simulink subsystem "hvb"  (R2020b)
settings: Solver=VariableStepAuto  StartTime=0.0  StopTime=10.0  RelTol=1e-3
undefined symbols (not defined in the file or in its folder): AmbTemp, batteryHV, DiscIntNeverNeededParam, hvBatterySOC_pct, motorDrive, nominalCapacity_kWh, packVoltage_V
libraries: fl_lib x14, nesl_utility x10, sdl_lib x1, ee_lib x1
settings Model: Creator=Dmitry  LastModifiedBy=Dmitry

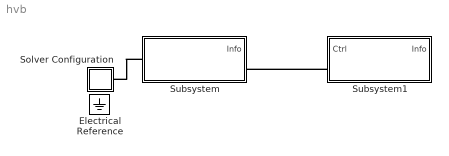
== system hvb ==
  Electrical Reference : fl_lib/Electrical/Electrical Elements/Electrical Reference
  Solver Configuration : Subsystem
      settings: PortSchema="{\"entries\":[{\"content\":{\"sides\":[{\"content\":{\"connectorIds\":[]},\"type\":\"ConnectorPlacement.EquallySpacedRectSide\",\"uuid\":\"4a7e26c2-e9e9-4fea-b605-533b1a682be7\"},{\"content\":{\"connectorIds\":[\"RConn1\"],\"side\":\"RIGHT\"},\"type\":\"ConnectorPlacement.EquallySpacedRectSide\",\"uuid\":\"0210e324-555e-4372-b836-fcc8ab23e933\"},{\"content\":{\"connectorIds\":[],\"side\":\"TOP\"},\"type\":\"ConnectorPlacement.EquallySpacedRectSide\",\"uuid\":\"9bbae011-e6fc-4534-a44f-d79a5697c939\"},{\"content\":{\"connectorIds\":[\"RConn2\"],\"side\":\"BOTTOM\"},\"type\":\"ConnectorPlacement.EquallySpacedRectSide\",\"uuid\":\"d5829c0a-26ea-402d-a1c6-900997ddf1a8\"}]},\"type\":\"ConnectorPlacement.EquallySpacedConnector\",\"uuid\":\"f4e17c65-54c6-42fe-a467-9c6b014b697a\"}],\"packageUris\":[\"http://schema.mathworks.com/mf0/Connector/19700101\"],\"version\":\"1.0\"}"
  Subsystem : Subsystem
  Subsystem1 : Subsystem
  connections:
  Subsystem/LConn1 -- Solver Configuration/RConn1
  Subsystem1/LConn1 -- Subsystem/RConn1

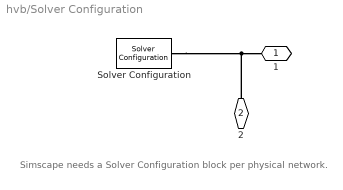
== system hvb/Solver Configuration ==
  note: Simscape needs a Solver Configuration block per physical network.
  Solver Configuration : nesl_utility/Solver Configuration  PhysicalDomain=network_engine_domain  SubClassName=solver  LeftPortType=input  RightPortType=generic  Tones=[]  Harmonics=[]  SimulateNoise=off  Profile=off  UseLocalSampling=off  EnableSwitchedLinearOptims=on  FrequencyDomain=off  UseCCode=off  RelTol=0.001  AbsTol=1e-06  MinStep=1e-09  ToWorkspace=off  RevertToSquareIcSolve=off  NumHomotopyIterations=100  PhasorMode=off  PhasorModeNumHarmonics=1  DoDC=off  ResidualTolerance=1e-6  UseLocalSolver=off  LocalSolverChoice=NE_BACKWARD_EULER_ADVANCER  LocalSolverSampleTime=0.01  DoFixedCost=off  MaxNonlinIter=3  MaxModeIter=2  ComputeImpulses=off  ImpulseIterations=2  LinearAlgebra=auto  EquationFormulation=NE_TIME_EF  DelaysMemoryBudget=1024  AutomaticFiltering=on  FilteringTimeConstant=0.001  PartitionStorageMethod=AS_NEEDED  PartitionMemoryBudget=1024  PartitionMethod=FAST
      settings: AttributesFormatString=Local solver %<UseLocalSolver>
  1 : PMIOPort  Side=Right
  2 : PMIOPort  Port=2  Side=Right
  connections:
  Solver Configuration/RConn1 -- 1/RConn1 -- 2/RConn1

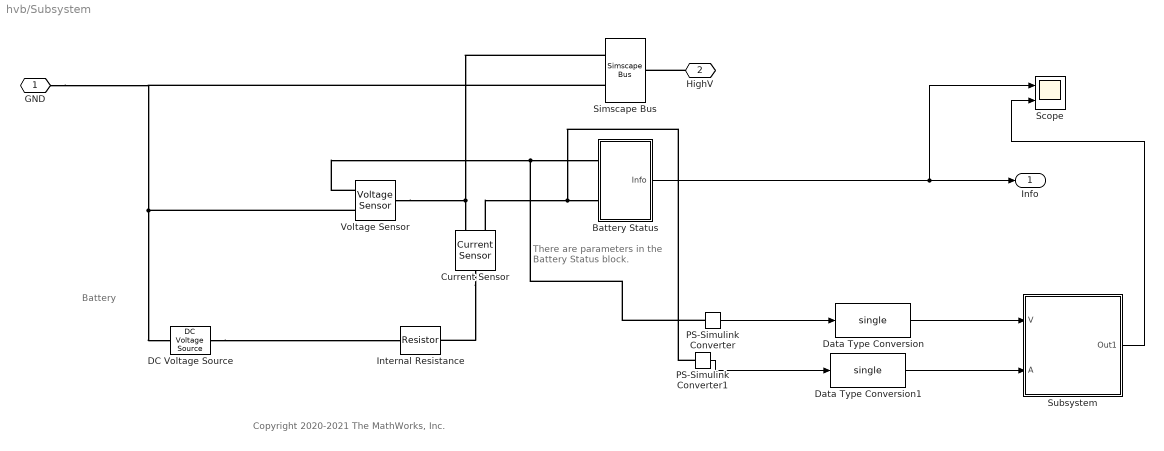
== system hvb/Subsystem ==
  note: Copyright 2020-2021 The MathWorks, Inc.
  note: There are parameters
      | in the Battery Status block.
  note: Battery
  Battery Status : Subsystem
  Current Sensor : fl_lib/Electrical/Electrical Sensors/Current Sensor
  DC Voltage Source : fl_lib/Electrical/Electrical Sources/DC Voltage Source  v0=batteryHV.packVoltage_V V
      settings: AttributesFormatString=%<v0> [%<v0_unit>]
  Data Type Conversion : DataTypeConversion  OutDataTypeStr=single
  Data Type Conversion1 : DataTypeConversion  OutDataTypeStr=single
  Internal Resistance : fl_lib/Electrical/Electrical Elements/Resistor  R=batteryHV.internal_R_Ohm Ohm  i_specify=off  i_priority=High  i=0 A  i_nominal_specify=off  i_nominal_unit=A  i_nominal_value=1  v_specify=off  v_priority=High  v=0 V  v_nominal_specify=off  v_nominal_unit=V  v_nominal_value=1
      settings: AttributesFormatString=%<R> [%<R_unit>]
  PS-Simulink Converter : nesl_utility/PS-Simulink Converter  PhysicalDomain=network_engine_domain  SubClassName=ps_output  LeftPortType=input  RightPortType=output  PseudoPeriodic=off  Frequencies=[]  Unit=inherit  AffineConversion=off
  PS-Simulink Converter1 : nesl_utility/PS-Simulink Converter  PhysicalDomain=network_engine_domain  SubClassName=ps_output  LeftPortType=input  RightPortType=output  PseudoPeriodic=off  Frequencies=[]  Unit=inherit  AffineConversion=off
  Scope : Scope  NumInputPorts=2
  Simscape Bus : SimscapeBus  HierarchyStrings=plus;minus
  Subsystem : Subsystem
  Voltage Sensor : fl_lib/Electrical/Electrical Sensors/Voltage Sensor
  GND : PMIOPort  Side=Left
  HighV : PMIOPort  Port=2  Side=Right
  Info : Outport
  wires:
  Data Type Conversion/1 -> Subsystem/1(V)
  PS-Simulink Converter1/1 -> Data Type Conversion1/1
  Battery Status/1(Info) -> Scope/1, Info/1
  Data Type Conversion1/1 -> Subsystem/2(A)
  PS-Simulink Converter/1 -> Data Type Conversion/1
  Subsystem/1(Out1) -> Scope/2
  connections:
  Voltage Sensor/RConn2 -- DC Voltage Source/RConn1 -- GND/RConn1 -- Simscape Bus/LConn2
  Simscape Bus/LConn1 -- Voltage Sensor/LConn1 -- Current Sensor/RConn2
  Current Sensor/RConn1 -- PS-Simulink Converter1/LConn1 -- Battery Status/LConn2
  Voltage Sensor/RConn1 -- PS-Simulink Converter/LConn1 -- Battery Status/LConn1
  HighV/RConn1 -- Simscape Bus/RConn1
  DC Voltage Source/LConn1 -- Internal Resistance/LConn1
  Current Sensor/LConn1 -- Internal Resistance/RConn1

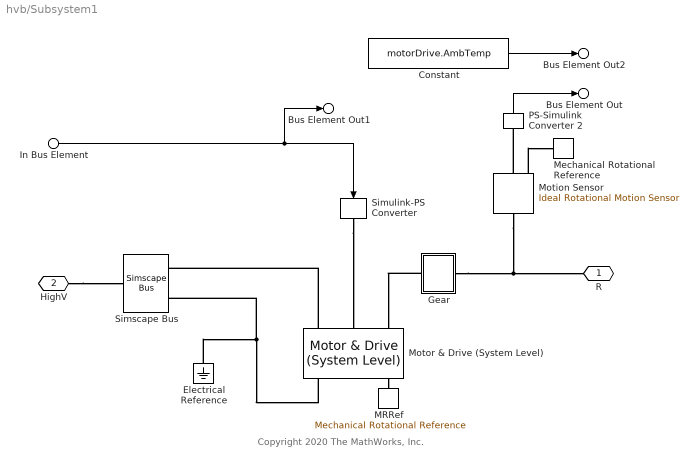
== system hvb/Subsystem1 ==
  note: Copyright 2020 The MathWorks, Inc.
  In Bus Element : Inport  PortName=Ctrl  Element=TorqueCmd
      settings: AttributesFormatString=%<Unit>
  " Simscape Bus" : SimscapeBus  HierarchyStrings=plus;minus
  Constant : Constant  Value=motorDrive.AmbTemp
  Electrical Reference : fl_lib/Electrical/Electrical Elements/Electrical Reference
  Gear : Subsystem
  MRRef : fl_lib/Mechanical/Rotational Elements/Mechanical Rotational Reference
  Mechanical Rotational Reference : fl_lib/Mechanical/Rotational Elements/Mechanical Rotational Reference
  Motion Sensor : fl_lib/Mechanical/Mechanical Sensors/Ideal Rotational Motion Sensor  wrap_angle=simscape.enum.onoff.off  offset=0 rad
  Motor & Drive (System Level) : ee_lib/Electromechanical/Motor & Drive (System Level)  torque_speed_param=2  overtorque_param=ee.enum.electromech.overtorque.no  T_t=[.09, .08, .07, 0] N*m  T_t_intermittent=[.36, .32, .28, 0] N*m  w_t=[0, 3750, 7500, 8000] rpm  torque_max=motorDrive.simplePmsmDrv_trqMax_Nm N*m  power_max=motorDrive.simplePmsmDrv_powMax_W W  torque_max_intermittent=0.4 N*m  power_max_intermittent=120 W  time_overtorque=30 s  time_recover=60 s  Tc=motorDrive.simplePmsmDrv_timeConst_s s  losses_param=2  eff=100  w_eff=3750 rpm  T_eff=0.08 N*m  Piron=0 W  Pbase=0 W  w_eff_vec=motorDrive.simplePmsmDrv_spdVec_rpm rpm  T_eff_vec=motorDrive.simplePmsmDrv_trqVec_Nm N*m  v_eff_vec=[100, 250, 400] V  losses_mat=motorDrive.simplePmsmDrv_LossTbl_W W  efficiency_mat=[95, 95, 95, 95; 95, 95, 95, 95; 95, 95, 95, 95; 95, 95, 95, 95; 95, 95, 95, 95]  losses_mat_3D=ones(5, 4, 3) W  efficiency_mat_3D=95 * ones(5, 4, 3)  Res=0 Ohm  J=motorDrive.simplePmsmDrv_rotorInertia_kg_m2 kg*m^2  lam=motorDrive.simplePmsmDrv_rotorDamping_Nm_per_radps N*m/(rad/s)  speed0=motorDrive.simplePmsmDrv_initialRotorSpd_rpm rpm  faulted_specify=off  faulted_priority=None  faulted=0  faulted_nominal_specify=off  faulted_nominal_unit=1  faulted_nominal_value=1  torqueLimitContinuous_specify=off  torqueLimitContinuous_priority=None  torqueLimitContinuous=0 N*m  torqueLimitContinuous_nominal_specify=off  torqueLimitContinuous_nominal_unit=N*m  torqueLimitContinuous_nominal_value=1  alpha=3.93e-3 1/K  Tmeas=25 degC  Tmeas2=125 degC  losses_mat_T2=[1.49, 1.74, 2.49, 3.74; .42, .67, 1.42, 2.67; .06, .31, 1.06, 2.31; .42, .67, 1.42, 2.67; 1.49, 1.74, 2.49, 3.74] W  efficiency_mat_T2=[95, 95, 95, 95; 95, 95, 95, 95; 95, 95, 95, 95; 95, 95, 95, 95; 95, 95, 95, 95]  losses_mat_3D_T2=ones(5, 4, 3) W  efficiency_mat_3D_T2=95 * ones(5, 4, 3)  thermal_mass=100 J/K  initial_temperature=25 degC  fault_condition=1  fault_threshold=0.5
      settings: SourceProductBaseCode=PS  LogSimulationData=on
  PS-Simulink Converter 2 : nesl_utility/PS-Simulink Converter  PhysicalDomain=network_engine_domain  SubClassName=ps_output  LeftPortType=input  RightPortType=output  PseudoPeriodic=off  Frequencies=[]  Unit=rpm  AffineConversion=off
  Simulink-PS Converter : nesl_utility/Simulink-PS Converter  PhysicalDomain=network_engine_domain  SubClassName=ps_input  LeftPortType=input  RightPortType=output  PseudoPeriodic=off  Frequencies=[]  NoiseDistribution=none  NoiseParameters=[]  Unit=N*m  AffineConversion=off  FilteringAndDerivatives=zero  SimscapeFilterOrder=1  InputFilterTimeConstant=.001  UdotUserProvided=0
  R : PMIOPort  Side=Right
  HighV : PMIOPort  Port=2  Side=Left
  Bus Element Out : Outport  PortName=Info  Element=MotorSpd
      settings: AttributesFormatString=%<Unit>
  Bus Element Out1 : Outport  PortName=Info  Element=TrqCmd
      settings: AttributesFormatString=%<Unit>
  Bus Element Out2 : Outport  PortName=Info  Element=Temp
      settings: AttributesFormatString=%<Unit>
  wires:
  In Bus Element/1 -> Bus Element Out1/1, Simulink-PS Converter/1
  PS-Simulink Converter 2/1 -> Bus Element Out/1
  Constant/1 -> Bus Element Out2/1
  connections:
  " Simscape Bus"/LConn2 -- Electrical Reference/LConn1 -- Motor & Drive (System Level)/RConn1
  Gear/RConn1 -- R/RConn1 -- Motion Sensor/LConn1
  Gear/LConn1 -- Motor & Drive (System Level)/LConn3
  Motion Sensor/RConn2 -- PS-Simulink Converter 2/LConn1
  HighV/RConn1 -- " Simscape Bus"/RConn1
  Motor & Drive (System Level)/LConn1 -- " Simscape Bus"/LConn1
  Motion Sensor/RConn1 -- Mechanical Rotational Reference/LConn1
  Motor & Drive (System Level)/RConn3 -- MRRef/LConn1
  Simulink-PS Converter/RConn1 -- Motor & Drive (System Level)/LConn2

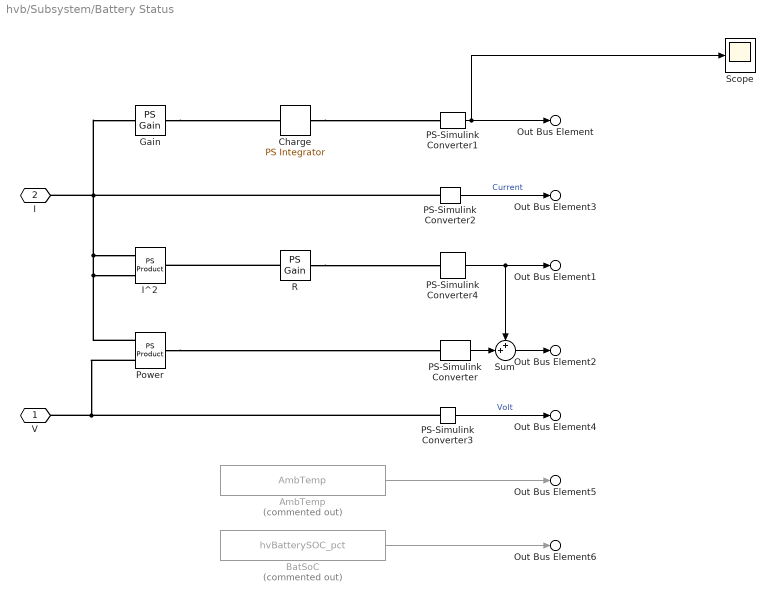
== system hvb/Subsystem/Battery Status ==
  AmbTemp : Constant  Commented=on  Value=AmbTemp
  BatSoC : Constant  Commented=on  Value=hvBatterySOC_pct
  Charge : fl_lib/Physical Signals/Linear Operators/PS Integrator  x0=initial.hvBatteryCharge_Ah A*hr
      settings: AttributesFormatString=%<x0> [%<x0_unit>]  SourceProductBaseCode=SS
  Gain : fl_lib/Physical Signals/Functions/PS Gain  gain=-1
      settings: AttributesFormatString=%<gain>
  I^2 : fl_lib/Physical Signals/Functions/PS Product
  PS-Simulink Converter : nesl_utility/PS-Simulink Converter  PhysicalDomain=network_engine_domain  SubClassName=ps_output  LeftPortType=input  RightPortType=output  PseudoPeriodic=off  Frequencies=[]  Unit=kW  AffineConversion=off
  PS-Simulink Converter1 : nesl_utility/PS-Simulink Converter  PhysicalDomain=network_engine_domain  SubClassName=ps_output  LeftPortType=input  RightPortType=output  PseudoPeriodic=off  Frequencies=[]  Unit=A*hr  AffineConversion=off
  PS-Simulink Converter2 : nesl_utility/PS-Simulink Converter  PhysicalDomain=network_engine_domain  SubClassName=ps_output  LeftPortType=input  RightPortType=output  PseudoPeriodic=off  Frequencies=[]  Unit=A  AffineConversion=off
  PS-Simulink Converter3 : nesl_utility/PS-Simulink Converter  PhysicalDomain=network_engine_domain  SubClassName=ps_output  LeftPortType=input  RightPortType=output  PseudoPeriodic=off  Frequencies=[]  Unit=V  AffineConversion=off
  PS-Simulink Converter4 : nesl_utility/PS-Simulink Converter  PhysicalDomain=network_engine_domain  SubClassName=ps_output  LeftPortType=input  RightPortType=output  PseudoPeriodic=off  Frequencies=[]  Unit=kW  AffineConversion=off
  Power : fl_lib/Physical Signals/Functions/PS Product
  R : fl_lib/Physical Signals/Functions/PS Gain  gain=batteryHV.internal_R_Ohm Ohm
      settings: AttributesFormatString=%<gain> [%<gain_unit>]
  Scope : Scope
  Sum : Sum  Inputs=++|
  V : PMIOPort  Side=Left
  I : PMIOPort  Port=2  Side=Left
  Out Bus Element : Outport  PortName=Info  Element=Charge
      settings: AttributesFormatString=%<Unit>
  Out Bus Element3 : Outport  PortName=Info  Element=Current
      settings: AttributesFormatString=%<Unit>
  Out Bus Element1 : Outport  PortName=Info  Element=PowerLoss
      settings: AttributesFormatString=%<Unit>
  Out Bus Element2 : Outport  PortName=Info  Element=Power
      settings: AttributesFormatString=%<Unit>
  Out Bus Element4 : Outport  PortName=Info  Element=Volt
      settings: AttributesFormatString=%<Unit>
  Out Bus Element5 : Outport  PortName=Info  Element=BatTemp
      settings: AttributesFormatString=%<Unit>
  Out Bus Element6 : Outport  PortName=Info  Element=BatSoC
      settings: AttributesFormatString=%<Unit>
  wires:
  PS-Simulink Converter4/1 -> Out Bus Element1/1, Sum/1
  PS-Simulink Converter1/1 -> Out Bus Element/1, Scope/1
  Sum/1 -> Out Bus Element2/1
  PS-Simulink Converter/1 -> Sum/2
  PS-Simulink Converter2/1 -> Out Bus Element3/1  "Current"
  PS-Simulink Converter3/1 -> Out Bus Element4/1  "Volt"
  AmbTemp/1 -> Out Bus Element5/1
  BatSoC/1 -> Out Bus Element6/1
  connections:
  R/RConn1 -- PS-Simulink Converter4/LConn1
  R/LConn1 -- I^2/RConn1
  PS-Simulink Converter2/LConn1 -- I/RConn1 -- Gain/LConn1 -- I^2/LConn2 -- Power/LConn2 -- I^2/LConn1
  Power/RConn1 -- PS-Simulink Converter/LConn1
  Charge/RConn1 -- PS-Simulink Converter1/LConn1
  Gain/RConn1 -- Charge/LConn1
  V/RConn1 -- PS-Simulink Converter3/LConn1 -- Power/LConn1

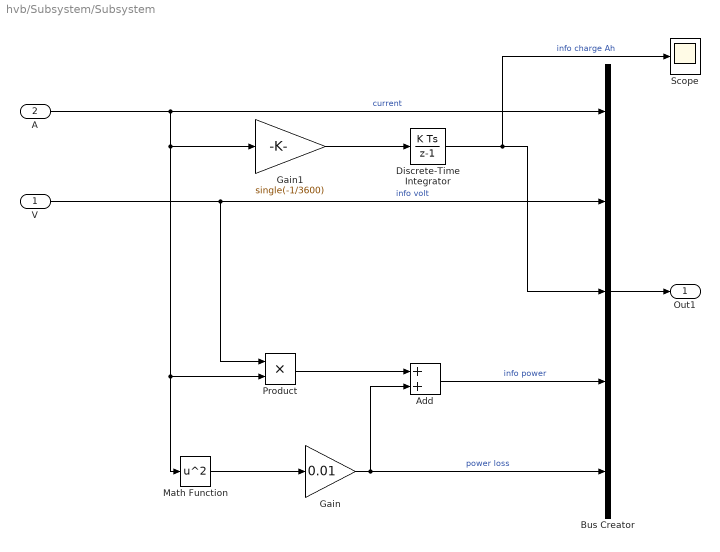
== system hvb/Subsystem/Subsystem ==
  V : Inport
  A : Inport  Port=2
  Add : Sum
  Bus Creator : BusCreator  Inputs=5  OutDataTypeStr=Bus: Bus
  Discrete-Time Integrator : DiscreteIntegrator  gainval=nominalCapacity_kWh/packVoltage_V*1000*hvBatterySOC_pct/100  InitialCondition=8  SampleTime=-1  OutDataTypeStr=single  ICPrevOutput=DiscIntNeverNeededParam  ICPrevScaledInput=DiscIntNeverNeededParam
  Gain : Gain  Gain=0.01
  Gain1 : Gain  Gain=single(-1/3600)
  Math Function : Math  Operator=square  SaturateOnIntegerOverflow=on
  Product : Product
  Scope : Scope
  Out1 : Outport  OutDataTypeStr=Bus: Bus
  wires:
  V/1 -> Bus Creator/2, Product/1  "info volt"
  Bus Creator/1 -> Out1/1
  Discrete-Time Integrator/1 -> Scope/1, Bus Creator/3  "info charge Ah"
  Math Function/1 -> Gain/1
  A/1 -> Math Function/1, Product/2, Gain1/1, Bus Creator/1  "current"
  Add/1 -> Bus Creator/4  "info power"
  Product/1 -> Add/1
  Gain/1 -> Add/2, Bus Creator/5  "power loss"
  Gain1/1 -> Discrete-Time Integrator/1

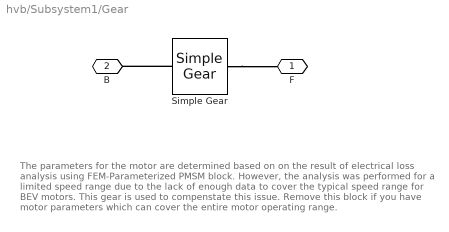
== system hvb/Subsystem1/Gear ==
  note: The parameters for the motor are determined based on on the result of electrical loss analysis using FEM-Parameterized PMSM block. However, the analysis was performed for a limited speed range due to the lack of enough data to cover the typical speed range for BEV motors. This gear is used to compenstate this issue. Remove this block if you have motor parameters which can cover the entire motor operating range.
  Simple Gear : sdl_lib/Gears/Simple Gear  ratio=motorDrive.gearRatioCompensation  rotation_direction=3-2*(1)  friction_model=sdl.enum.gear_efficiencies_load.off  mu_visc=[0, 0] N*m/(rad/s)  T_noload=0.1 N*m  T_nom=5 N*m  efficiency_nom=0.8  efficiency=0.8  temperature_TLU=[280, 300, 320] K  load_TLU=[1, 5, 10] N*m  efficiency_TLU=[.95, .9, .85]  efficiency_TLU2=[.85, .8, .75; .95, .9, .85; .85, .8, .7]  w_thr=0.01 rad/s  pwr_thr=0.001 W  thermal_mass=50 J/K  enable_faults=simscape.enum.onoff.off  efficiency_fault=0.05  external_fault=simscape.enum.onoff.off  temporal_fault=simscape.enum.onoff.off  fault_time=5 s  fault_angles=pi / 12 rad  report_fault=(1)-1  temperature_specify=off  temperature_priority=High  temperature=300 K  temperature_nominal_specify=off  temperature_nominal_unit=K  temperature_nominal_value=1
      settings: AttributesFormatString=%<ratio>
  F : PMIOPort  Side=Right
  B : PMIOPort  Port=2  Side=Left
  connections:
  Simple Gear/RConn1 -- F/RConn1
  Simple Gear/LConn1 -- B/RConn1
